simulink model "copi_Customtimer"  (R2025b)
settings: Solver=VariableStepAuto  StartTime=0.0  StopTime=20  RelTol=1e-3
libraries: dspsigops x1
settings Model: Creator=Antonio  LastModifiedBy=Antonio

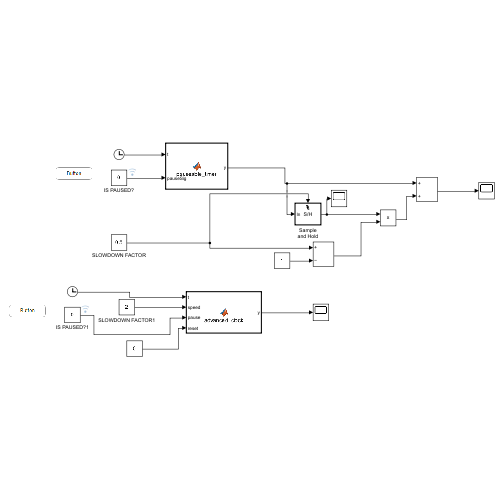
[thumbnail: Simulink's stored preview of the top-level diagram]
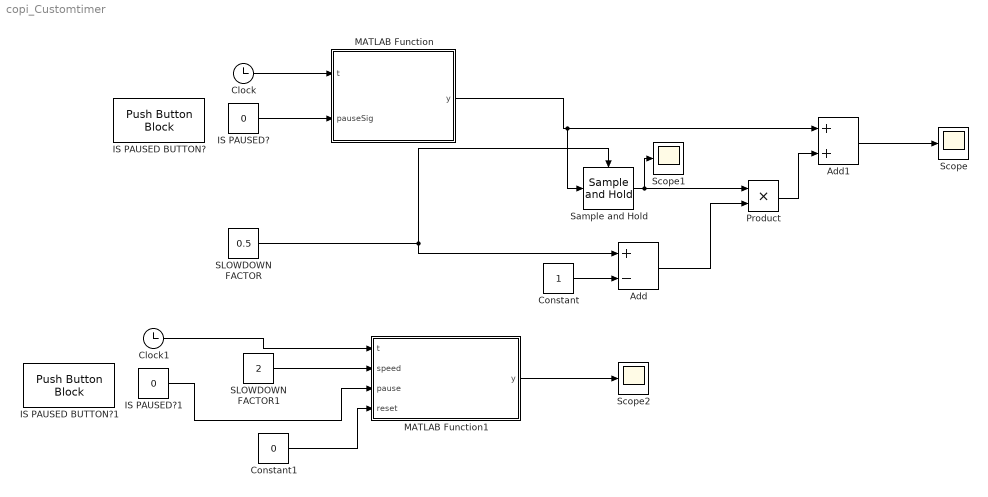
== system copi_Customtimer ==
  Add : Sum  Inputs=+-
  Add1 : Sum
  Clock : Clock
  Clock1 : Clock
  Constant : Constant
  Constant1 : Constant  Value=0
  IS PAUSED BUTTON? : PushButtonBlock  ButtonType=Latch  IconOnColor=[0.0, 0.39215686274509803, 0.0]  IconOffColor=[0.0, 1.0, 0.0]  OffValue=0.000000
  IS PAUSED BUTTON?1 : PushButtonBlock  ButtonType=Latch  IconOnColor=[0.0, 0.39215686274509803, 0.0]  IconOffColor=[0.0, 1.0, 0.0]  OffValue=0.000000
  IS PAUSED? : Constant  Value=0
  IS PAUSED?1 : Constant  Value=0
  MATLAB Function : MATLAB Function  TreatAsAtomicUnit=on
  MATLAB Function1 : MATLAB Function  TreatAsAtomicUnit=on
  Product : Product
  SLOWDOWN FACTOR : Constant  Value=0.5
  SLOWDOWN FACTOR1 : Constant  Value=2
  Sample and Hold : dspsigops/Sample and Hold  trig=Falling edge  initCond=0  latchinput=off
  Scope : Scope
      settings: ActiveDisplayYMinimum=-4.2683249723173073  ActiveDisplayYMaximum=19.036883445445014
  Scope1 : Scope
      settings: ActiveDisplayYMinimum=-1  ActiveDisplayYMaximum=1
  Scope2 : Scope
      settings: ActiveDisplayYMinimum=-4.2683249723173073  ActiveDisplayYMaximum=19.036883445445014  DataLoggingVariableName=ScopeData2
  wires:
  Clock/1 -> MATLAB Function/1(t)
  IS PAUSED?/1 -> MATLAB Function/2(pauseSig)
  SLOWDOWN FACTOR/1 -> Sample and Hold/Trigger, Add/1
  Constant/1 -> Add/2
  Add/1 -> Product/2
  MATLAB Function/1(y) -> Sample and Hold/1, Add1/1
  Product/1 -> Add1/2
  Add1/1 -> Scope/1
  Sample and Hold/1 -> Scope1/1, Product/1
  SLOWDOWN FACTOR1/1 -> MATLAB Function1/2(speed)
  MATLAB Function1/1(y) -> Scope2/1
  Clock1/1 -> MATLAB Function1/1(t)
  IS PAUSED?1/1 -> MATLAB Function1/3(pause)
  Constant1/1 -> MATLAB Function1/4(reset)

== matlab function copi_Customtimer/MATLAB Function1 ==
  data: t input; y output; speed input; pause input; reset input
function y = advanced_clock(t, speed, pause, reset)

persistent last_t scaled_time initialized

if isempty(initialized) || reset
    last_t = t;
    scaled_time = 0;
    initialized = true;
end

dt = t - last_t;

if speed <= 0
    speed = 1;
end

if ~pause
    scaled_time = scaled_time + dt * speed;
end

y = scaled_time;

last_t = t;

== matlab function copi_Customtimer/MATLAB Function ==
  data: t input; y output; pauseSig input
function y= pauseable_timer(t, pauseSig)
% t        : simulation time from Clock
% pauseSig : 1 = pause, 0 = run
% y        : net elapsed time

persistent startTime totalPaused pauseStart wasPaused frozenValue initialized

%Only do this first loop
if isempty(initialized)
    startTime   = t;
    totalPaused = 0;
    pauseStart  = 0;
    wasPaused   = false;
    frozenValue = 0;
    initialized = true;
end

if pauseSig ~= 0
    % Entering pause
    if ~wasPaused
        pauseStart  = t;
        frozenValue = t - startTime - totalPaused;
        wasPaused   = true;
    end
    
    % Hold the output constant while paused
    y = frozenValue;
else
    % Leaving pause
    if wasPaused
        totalPaused = totalPaused + (t - pauseStart);
        wasPaused   = false;
    end
    
    % Normal running output
    y = t - startTime - totalPaused;
end
